simulink model "GainSchedulingSimulink"  (R2023b)
settings: Solver=VariableStepAuto  StartTime=0.0  StopTime=50.0  RelTol=1e-3
undefined symbols (not defined in the file): r, w0, zeta
settings Model: Creator=beniaminosquitieri  LastModifiedBy=beniaminosquitieri

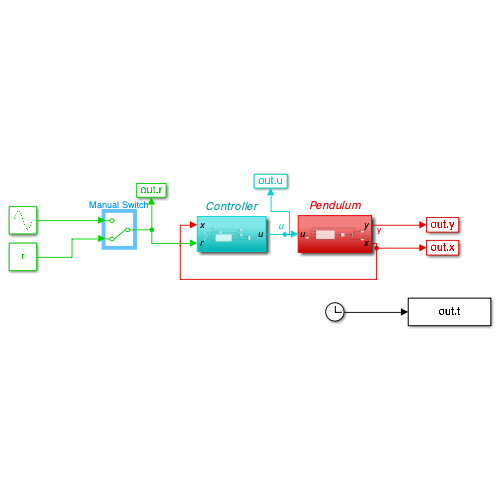
[thumbnail: Simulink's stored preview of the top-level diagram]
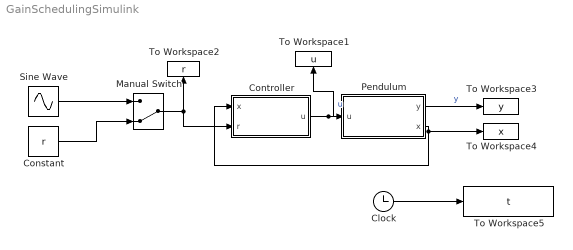
== system GainSchedulingSimulink ==
  Clock : Clock
  Constant : Constant  Value=r
  Controller : Subsystem
  Manual Switch : ManualSwitch  CurrentSetting=0
  Pendulum : Subsystem
  Sine Wave : Sin  Amplitude=0.5  Frequency=0.1  SampleTime=0
  To Workspace1 : ToWorkspace  VariableName=u  SaveFormat=Timeseries  SampleTime=-1
  To Workspace2 : ToWorkspace  VariableName=r  SaveFormat=Timeseries  SampleTime=-1
  To Workspace3 : ToWorkspace  VariableName=y  SaveFormat=Timeseries  SampleTime=-1
  To Workspace4 : ToWorkspace  VariableName=x  SaveFormat=Timeseries  SampleTime=-1
  To Workspace5 : ToWorkspace  VariableName=t  SaveFormat=Timeseries  SampleTime=-1
  wires:
  Manual Switch/1 -> Controller/2(r), To Workspace2/1
  Pendulum/1(y) -> To Workspace3/1  "y"
  Controller/1(u) -> To Workspace1/1, Pendulum/1(u)  "u"
  Pendulum/2(x) -> Controller/1(x), To Workspace4/1
  Sine Wave/1 -> Manual Switch/1
  Constant/1 -> Manual Switch/2
  Clock/1 -> To Workspace5/1

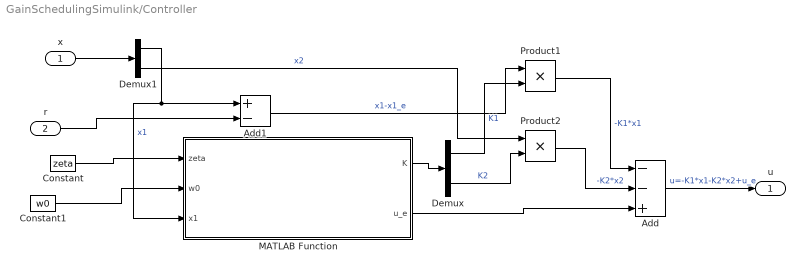
== system GainSchedulingSimulink/Controller ==
  x : Inport
  r : Inport  Port=2
  Add : Sum  Inputs=--+
  Add1 : Sum  Inputs=+-
  Constant : Constant  Value=zeta
  Constant1 : Constant  Value=w0
  Demux : Demux  Outputs=2
  Demux1 : Demux  Outputs=2
  MATLAB Function : MATLAB Function  TreatAsAtomicUnit=on
  Product1 : Product
  Product2 : Product
  u : Outport
  wires:
  Demux/1 -> Product1/2  "K1"
  Constant/1 -> MATLAB Function/1(zeta)
  Constant1/1 -> MATLAB Function/2(w0)
  Demux/2 -> Product2/2  "K2"
  Product2/1 -> Add/2  "-K2*x2"
  Product1/1 -> Add/1  "-K1*x1"
  MATLAB Function/1(K) -> Demux/1
  Add1/1 -> Product1/1  "x1-x1_e"
  x/1 -> Demux1/1
  Demux1/1 -> Add1/1, MATLAB Function/3(x1)  "x1"
  Demux1/2 -> Product2/1  "x2"
  r/1 -> Add1/2
  Add/1 -> u/1  "u=-K1*x1-K2*x2+u_e"
  MATLAB Function/2(u_e) -> Add/3

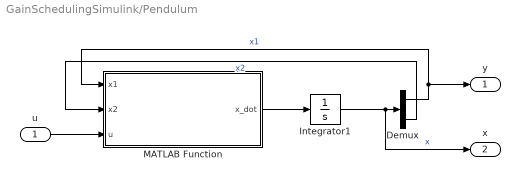
== system GainSchedulingSimulink/Pendulum ==
  u : Inport
  Demux : Demux  Outputs=2
  Integrator1 : Integrator  InitialCondition=0.0
  MATLAB Function : MATLAB Function  TreatAsAtomicUnit=on
  y : Outport
  x : Outport  Port=2
  wires:
  MATLAB Function/1(x_dot) -> Integrator1/1
  u/1 -> MATLAB Function/3(u)
  Integrator1/1 -> x/1, Demux/1  "x"
  Demux/1 -> MATLAB Function/1(x1), y/1  "x1"
  Demux/2 -> MATLAB Function/2(x2)  "x2"

== matlab function GainSchedulingSimulink/Controller/MATLAB Function ==
  data: K output; zeta input; w0 input; x1 input; u_e output
function [K,u_e] = compute_gains(zeta, w0, x1)

    K2 = 2*zeta*w0-1/10;
    K1 = w0^2+9.81*cos(x1);
    u_e=-9.81*sin(x1);
   
    K = [K1 K2];
    
end

== matlab function GainSchedulingSimulink/Pendulum/MATLAB Function ==
  data: x1 input; x_dot output; x2 input; u input
function x_dot= pendulum_plant(x1, x2, u)

    m = 1; 
    l = 1;
    b = 0.1;
    g = 9.81;
    
    x1_dot = x2;
    x2_dot = (g/l)*sin(x1) - (b/(m*l^2)*x2) + (u/(m*l^2));
    x_dot=[x1_dot,x2_dot];
       
end
